simulink model "flightcontroller"  (R2017b)
settings: Solver=FixedStepAuto  StartTime=0.0  StopTime=10.0  FixedStep=interval  RelTol=1e-3
values from neighbouring files (symbols this model uses):
  idle = 0    [Motor_Parameters.m]
settings Model: Creator=DanAdmin  LastModifiedBy=schapman

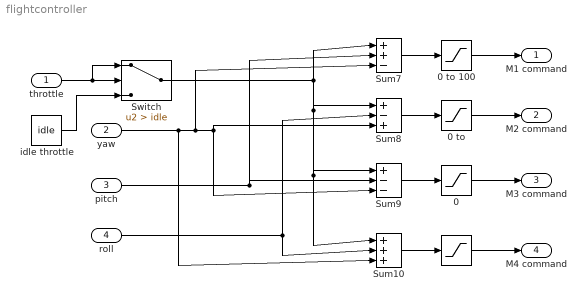
== system flightcontroller ==
  throttle : Inport
  yaw : Inport  Port=2
  pitch : Inport  Port=3
  roll : Inport  Port=4
  " " : Saturate  UpperLimit=100  LowerLimit=0
  "0  " : Saturate  UpperLimit=100  LowerLimit=0
  "0 to " : Saturate  UpperLimit=100  LowerLimit=0
  0 to 100 : Saturate  UpperLimit=100  LowerLimit=0
  Sum10 : Sum  Inputs=|+++
  Sum7 : Sum  Inputs=|++-
  Sum8 : Sum  Inputs=|+-+
  Sum9 : Sum  Inputs=|+--
  Switch : Switch  Criteria=u2 > Threshold  Threshold=idle
  idle throttle : Constant  Value=idle
  M1 command : Outport
  M2 command : Outport  Port=2
  M3 command : Outport  Port=3
  M4 command : Outport  Port=4
  wires:
  yaw/1 -> Sum7/3, Sum8/3, Sum9/3, Sum10/3
  Switch/1 -> Sum10/1, Sum9/1, Sum8/1, Sum7/1
  roll/1 -> Sum8/2, Sum10/2
  pitch/1 -> Sum9/2, Sum7/2
  Sum7/1 -> 0 to 100/1
  Sum9/1 -> "0  "/1
  Sum8/1 -> "0 to "/1
  Sum10/1 -> " "/1
  0 to 100/1 -> M1 command/1
  " "/1 -> M4 command/1
  "0  "/1 -> M3 command/1
  "0 to "/1 -> M2 command/1
  throttle/1 -> Switch/2, Switch/1
  idle throttle/1 -> Switch/3
